simulink model "robot_portique_2_axes"  (R2024b)
settings: Solver=VariableStepAuto  StartTime=0.0  StopTime=21  RelTol=1e-3
settings Model: Creator=firas  LastModifiedBy=firas

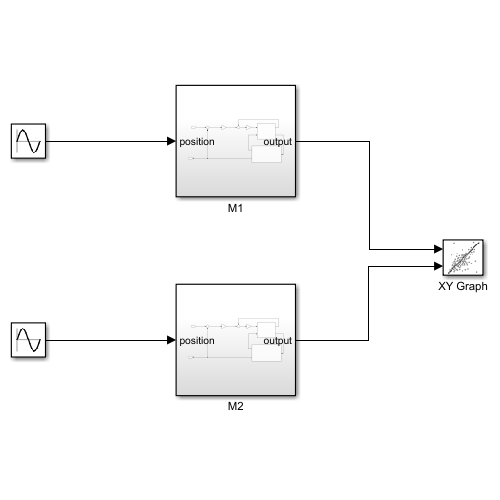
[thumbnail: Simulink's stored preview of the top-level diagram]
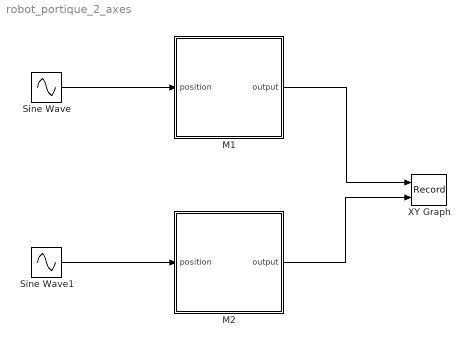
== system robot_portique_2_axes ==
  M1 : Subsystem
  M2 : Subsystem
  Sine Wave : Sin  Frequency=pi/10  Phase=pi/2  SampleTime=0
  Sine Wave1 : Sin  Frequency=pi/10  SampleTime=0
  XY Graph : Record  FileSettingsInternal="{\"entries\":[{\"content\":{\"excelSettings\":{\"content\":{},\"type\":\"Streamout.ExcelSettings\"}},\"type\":\"Streamout.FileSettingStorage\",\"uuid\":\"\"}],\"packageUris\":[\"http:\\/\\/schema.mathworks.com\\/mf0\\/streamout_blocks\\/R2020a\"],\"version\":\"1.0\"}"  Layout=[1 1]  SignalsInternal="{\"entries\":[{\"content\":{\"signals\":[{\"content\":{\"blockPath\":[],\"dimensions\":[1],\"domain\":\"\",\"lineColor\":\"#a2142f\",\"plots\":[ 1 ],\"port\":1,\"sid\":[\"\"],\"signalID\":1,\"signalName\":\"M1\"},\"type\":\"RecordBlkView.Signal\",\"uuid\":\"\"},{\"content\":{\"blockPath\":[],\"dimensions\":[1],\"domain\":\"\",\"lineColor\":\"#139fff\",\"plots\":[ 1 ],\"port\":2,\"sid\":[\"\"],\"signalID\":2,\"signalName\":\"M2\"},\"type\":\"RecordBlkView.Signal\",\"uuid\":\"\"}]},\"type\":\"RecordBlkView.InputSignals\",\"uuid\":\"\"}],\"packageUris\":[\"http:\\/\\/schema.mathworks.com\\/mf0\\/streamout_blocks\\/R2020a\"],\"version\":\"1.0\"}"  VisualizationBindings="{\"xyplotplugin\":{\"info\":[{\"series\":[{\"bindingParametersList\":[{\"parameter\":\"X-Axis\",\"signalID\":1,\"signalName\":\"M1\"},{\"parameter\":\"Y-Axis\",\"signalID\":2,\"signalName\":\"M2\"}],\"seriesID\":0}],\"subplotID\":1}]}}"  CompatibilityTag=XY
  wires:
  Sine Wave/1 -> M1/1(position)
  Sine Wave1/1 -> M2/1(position)
  M1/1(output) -> XY Graph/1
  M2/1(output) -> XY Graph/2

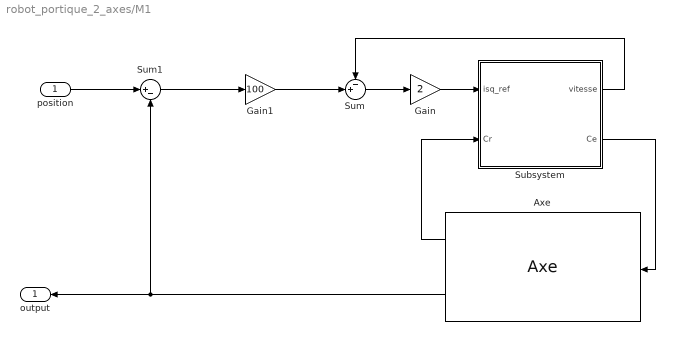
== system robot_portique_2_axes/M1 ==
  position : Inport
  Axe : S-Function  FunctionName=Axe  SFunctionModules=Axe_wrapper.c  SFunctionDeploymentMode=off  EnableBusSupport=off  mask(S-Function Builder){}
      mask help: Simulink:masks:SFunctionBuilder_MD
      mask init:
      | val = [[.9  0.75 0.75 1 1 .9 .9 1]',[1 1 0.75 0.75 .9 .9 1 .9]'];try , sys = get_param(gcb,'SfunBuilderFcnName');if isempty(sys), sys = get_param(gcb,'FunctionName'); end,catch, sys = get_param(gcb,'FunctionName'); end
      settings: CopyFcn=set_param(gcbh,'LinkStatus','none')  OpenFcn=sfunctionwizard(gcbh)
      mask Display:
      | plot(val(:,1),val(:,2))
      | disp(sys)
      | port_label('input',1,sprintf('%s', 'couple\_moteur'),'interpreter','tex')
      | port_label('output',1,sprintf('%s', 'couple\_resistant'),'interpreter','tex')
      | port_label('output',2,sprintf('%s', 'position'),'interpreter','tex')
  Gain : Gain  Gain=2
  Gain1 : Gain  Gain=100
  Subsystem : Subsystem
  Sum : Sum  Inputs=-+|
  Sum1 : Sum  Inputs=|+-
  output : Outport
  wires:
  Subsystem/1(vitesse) -> Sum/1
  Sum1/1 -> Gain1/1
  Axe/2 -> output/1, Sum1/2
  Gain1/1 -> Sum/2
  Subsystem/2(Ce) -> Axe/1
  Gain/1 -> Subsystem/1(isq_ref)
  Axe/1 -> Subsystem/2(Cr)
  Sum/1 -> Gain/1
  position/1 -> Sum1/1

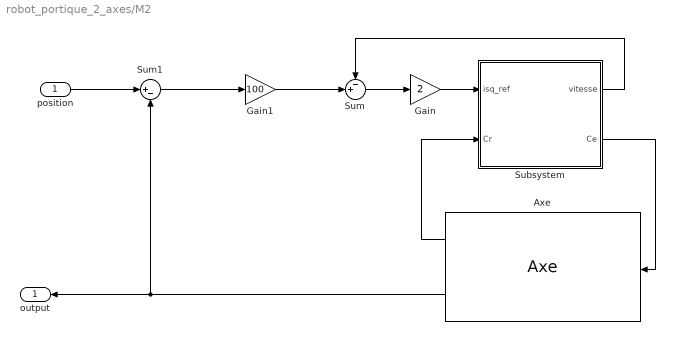
== system robot_portique_2_axes/M2 ==
  position : Inport
  Axe : S-Function  FunctionName=Axe  SFunctionModules=Axe_wrapper.c  SFunctionDeploymentMode=off  EnableBusSupport=off  mask(S-Function Builder){}
      mask help: Simulink:masks:SFunctionBuilder_MD
      mask init: same as robot_portique_2_axes/M1/Axe
      settings: CopyFcn=set_param(gcbh,'LinkStatus','none')  OpenFcn=sfunctionwizard(gcbh)
      mask Display:
      | plot(val(:,1),val(:,2))
      | disp(sys)
      | port_label('input',1,sprintf('%s', 'couple\_moteur'),'interpreter','tex')
      | port_label('output',1,sprintf('%s', 'couple\_resistant'),'interpreter','tex')
      | port_label('output',2,sprintf('%s', 'position'),'interpreter','tex')
  Gain : Gain  Gain=2
  Gain1 : Gain  Gain=100
  Subsystem : Subsystem
  Sum : Sum  Inputs=-+|
  Sum1 : Sum  Inputs=|+-
  output : Outport
  wires:
  position/1 -> Sum1/1
  Sum/1 -> Gain/1
  Axe/1 -> Subsystem/2(Cr)
  Gain/1 -> Subsystem/1(isq_ref)
  Subsystem/2(Ce) -> Axe/1
  Gain1/1 -> Sum/2
  Axe/2 -> Sum1/2, output/1
  Sum1/1 -> Gain1/1
  Subsystem/1(vitesse) -> Sum/1

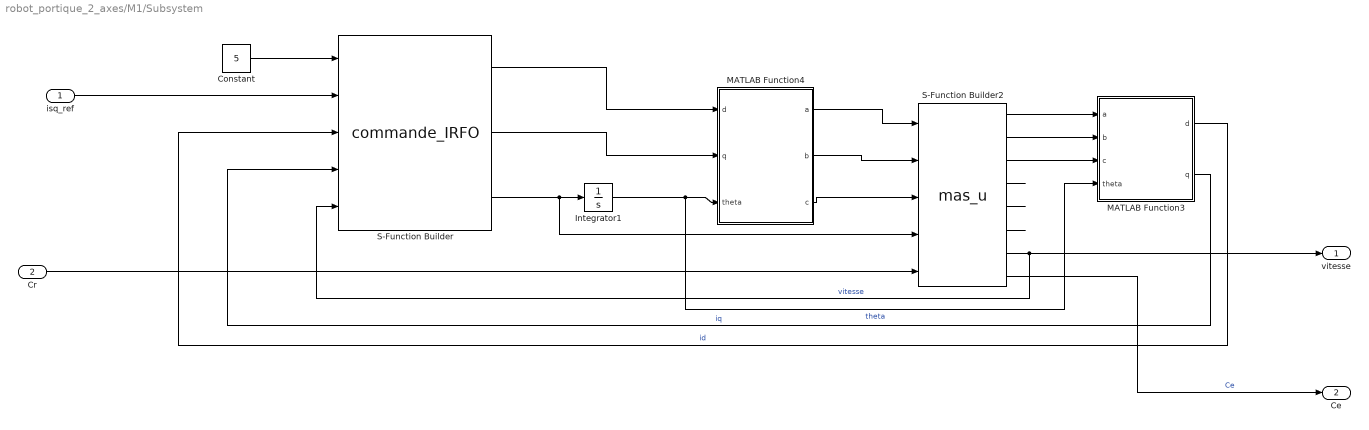
== system robot_portique_2_axes/M1/Subsystem ==
  isq_ref : Inport
  Cr : Inport  Port=2
  Constant : Constant  Value=5
  Integrator1 : Integrator
  MATLAB Function3 : MATLAB Function  TreatAsAtomicUnit=on
  MATLAB Function4 : MATLAB Function  TreatAsAtomicUnit=on
  S-Function Builder : S-Function  FunctionName=commande_IRFO  SFunctionModules=commande_IRFO_wrapper.c  SFunctionDeploymentMode=off  EnableBusSupport=off  mask(S-Function Builder){}
      mask help: Simulink:masks:SFunctionBuilder_MD
      mask init: same as robot_portique_2_axes/M1/Axe
      settings: CopyFcn=set_param(gcbh,'LinkStatus','none')  OpenFcn=sfunctionwizard(gcbh)
      mask Display:
      | plot(val(:,1),val(:,2))
      | disp(sys)
      | port_label('input',1,sprintf('%s', 'iphi\_ref'),'interpreter','tex')
      | port_label('input',2,sprintf('%s', 'isq\_ref'),'interpreter','tex')
      | port_label('input',3,sprintf('%s', 'isd'),'interpreter','tex')
      | port_label('input',4,sprintf('%s', 'isq'),'interpreter','tex')
      | port_label('input',5,sprintf('%s', 'vitesse'),'interpreter','tex')
      | port_label('output',1,sprintf('%s', 'vsd'),'interpreter','tex')
      | port_label('output',2,sprintf('%s', 'vsq'),'interpreter','tex')
      | port_label('output',3,sprintf('%s', 'ws'),'interpreter','tex')
  S-Function Builder2 : S-Function  FunctionName=mas_u  SFunctionModules=mas_u_wrapper.c  SFunctionDeploymentMode=off  EnableBusSupport=off  mask(S-Function Builder){}
      mask help: Simulink:masks:SFunctionBuilder_MD
      mask init: same as robot_portique_2_axes/M1/Axe
      settings: CopyFcn=set_param(gcbh,'LinkStatus','none')  OpenFcn=sfunctionwizard(gcbh)
      mask Display:
      | plot(val(:,1),val(:,2))
      | disp(sys)
      | port_label('input',1,sprintf('%s', 'vsa'),'interpreter','tex')
      | port_label('input',2,sprintf('%s', 'vsb'),'interpreter','tex')
      | port_label('input',3,sprintf('%s', 'vsc'),'interpreter','tex')
      | port_label('input',4,sprintf('%s', 'ws'),'interpreter','tex')
      | port_label('input',5,sprintf('%s', 'Cr'),'interpreter','tex')
      | port_label('output',1,sprintf('%s', 'isa'),'interpreter','tex')
      | port_label('output',2,sprintf('%s', 'isb'),'interpreter','tex')
      | port_label('output',3,sprintf('%s', 'isc'),'interpreter','tex')
      | port_label('output',4,sprintf('%s', 'ira'),'interpreter','tex')
      | port_label('output',5,sprintf('%s', 'irb'),'interpreter','tex')
      | port_label('output',6,sprintf('%s', 'irc'),'interpreter','tex')
      | port_label('output',7,sprintf('%s', 'vitesse'),'interpreter','tex')
      | port_label('output',8,sprintf('%s', 'Ce'),'interpreter','tex')
  vitesse : Outport
  Ce : Outport  Port=2
  wires:
  S-Function Builder2/4 -> ?
  S-Function Builder/2 -> MATLAB Function4/2(q)
  Integrator1/1 -> MATLAB Function4/3(theta), MATLAB Function3/4(theta)  "theta"
  S-Function Builder2/5 -> ?
  S-Function Builder/3 -> S-Function Builder2/4, Integrator1/1
  S-Function Builder2/1 -> MATLAB Function3/1(a)
  S-Function Builder2/7 -> vitesse/1, S-Function Builder/5  "vitesse"
  MATLAB Function3/1(d) -> S-Function Builder/3  "id"
  S-Function Builder2/2 -> MATLAB Function3/2(b)
  MATLAB Function4/1(a) -> S-Function Builder2/1
  S-Function Builder2/3 -> MATLAB Function3/3(c)
  Cr/1 -> S-Function Builder2/5
  MATLAB Function4/3(c) -> S-Function Builder2/3
  Constant/1 -> S-Function Builder/1
  S-Function Builder/1 -> MATLAB Function4/1(d)
  MATLAB Function3/2(q) -> S-Function Builder/4  "iq"
  MATLAB Function4/2(b) -> S-Function Builder2/2
  isq_ref/1 -> S-Function Builder/2
  S-Function Builder2/6 -> ?
  S-Function Builder2/8 -> Ce/1  "Ce"

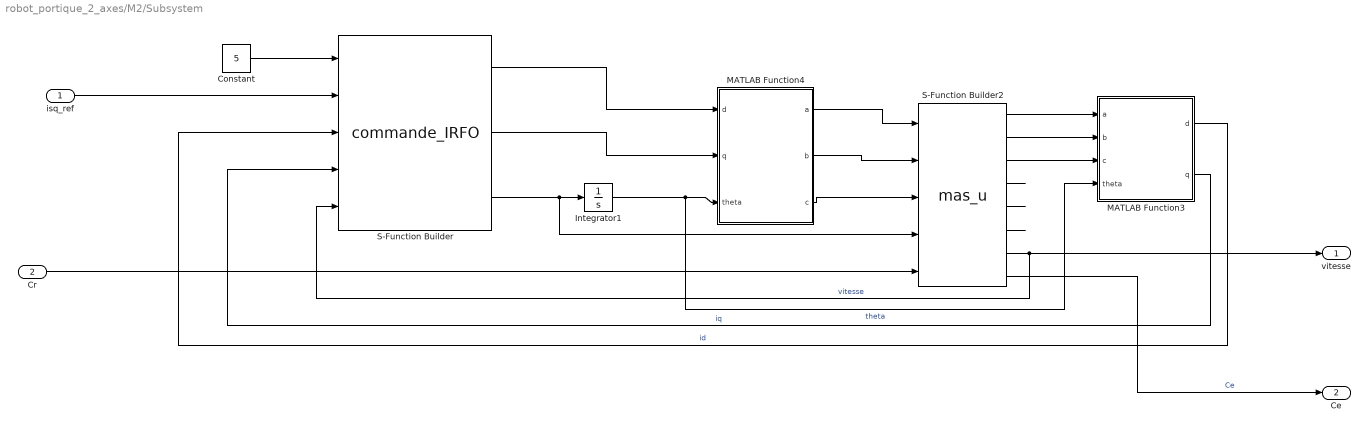
== system robot_portique_2_axes/M2/Subsystem ==
  isq_ref : Inport
  Cr : Inport  Port=2
  Constant : Constant  Value=5
  Integrator1 : Integrator
  MATLAB Function3 : MATLAB Function  TreatAsAtomicUnit=on
  MATLAB Function4 : MATLAB Function  TreatAsAtomicUnit=on
  S-Function Builder : S-Function  FunctionName=commande_IRFO  SFunctionModules=commande_IRFO_wrapper.c  SFunctionDeploymentMode=off  EnableBusSupport=off  mask(S-Function Builder){}
      mask help: Simulink:masks:SFunctionBuilder_MD
      mask init: same as robot_portique_2_axes/M1/Axe
      settings: CopyFcn=set_param(gcbh,'LinkStatus','none')  OpenFcn=sfunctionwizard(gcbh)
      mask Display:
      | plot(val(:,1),val(:,2))
      | disp(sys)
      | port_label('input',1,sprintf('%s', 'iphi\_ref'),'interpreter','tex')
      | port_label('input',2,sprintf('%s', 'isq\_ref'),'interpreter','tex')
      | port_label('input',3,sprintf('%s', 'isd'),'interpreter','tex')
      | port_label('input',4,sprintf('%s', 'isq'),'interpreter','tex')
      | port_label('input',5,sprintf('%s', 'vitesse'),'interpreter','tex')
      | port_label('output',1,sprintf('%s', 'vsd'),'interpreter','tex')
      | port_label('output',2,sprintf('%s', 'vsq'),'interpreter','tex')
      | port_label('output',3,sprintf('%s', 'ws'),'interpreter','tex')
  S-Function Builder2 : S-Function  FunctionName=mas_u  SFunctionModules=mas_u_wrapper.c  SFunctionDeploymentMode=off  EnableBusSupport=off  mask(S-Function Builder){}
      mask help: Simulink:masks:SFunctionBuilder_MD
      mask init: same as robot_portique_2_axes/M1/Axe
      settings: CopyFcn=set_param(gcbh,'LinkStatus','none')  OpenFcn=sfunctionwizard(gcbh)
      mask Display:
      | plot(val(:,1),val(:,2))
      | disp(sys)
      | port_label('input',1,sprintf('%s', 'vsa'),'interpreter','tex')
      | port_label('input',2,sprintf('%s', 'vsb'),'interpreter','tex')
      | port_label('input',3,sprintf('%s', 'vsc'),'interpreter','tex')
      | port_label('input',4,sprintf('%s', 'ws'),'interpreter','tex')
      | port_label('input',5,sprintf('%s', 'Cr'),'interpreter','tex')
      | port_label('output',1,sprintf('%s', 'isa'),'interpreter','tex')
      | port_label('output',2,sprintf('%s', 'isb'),'interpreter','tex')
      | port_label('output',3,sprintf('%s', 'isc'),'interpreter','tex')
      | port_label('output',4,sprintf('%s', 'ira'),'interpreter','tex')
      | port_label('output',5,sprintf('%s', 'irb'),'interpreter','tex')
      | port_label('output',6,sprintf('%s', 'irc'),'interpreter','tex')
      | port_label('output',7,sprintf('%s', 'vitesse'),'interpreter','tex')
      | port_label('output',8,sprintf('%s', 'Ce'),'interpreter','tex')
  vitesse : Outport
  Ce : Outport  Port=2
  wires:
  S-Function Builder2/8 -> Ce/1  "Ce"
  S-Function Builder2/6 -> ?
  isq_ref/1 -> S-Function Builder/2
  MATLAB Function4/2(b) -> S-Function Builder2/2
  MATLAB Function3/2(q) -> S-Function Builder/4  "iq"
  S-Function Builder/1 -> MATLAB Function4/1(d)
  Constant/1 -> S-Function Builder/1
  MATLAB Function4/3(c) -> S-Function Builder2/3
  Cr/1 -> S-Function Builder2/5
  S-Function Builder2/3 -> MATLAB Function3/3(c)
  MATLAB Function4/1(a) -> S-Function Builder2/1
  S-Function Builder2/2 -> MATLAB Function3/2(b)
  MATLAB Function3/1(d) -> S-Function Builder/3  "id"
  S-Function Builder2/7 -> S-Function Builder/5, vitesse/1  "vitesse"
  S-Function Builder2/1 -> MATLAB Function3/1(a)
  S-Function Builder/3 -> Integrator1/1, S-Function Builder2/4
  S-Function Builder2/5 -> ?
  Integrator1/1 -> MATLAB Function3/4(theta), MATLAB Function4/3(theta)  "theta"
  S-Function Builder/2 -> MATLAB Function4/2(q)
  S-Function Builder2/4 -> ?

== matlab function robot_portique_2_axes/M2/Subsystem/MATLAB Function3 ==
  data: a input; d output; b input; c input; theta input; q output
function [d,q] = Park_direct(a,b,c,theta)
    
     d = sqrt(2/3)*[cos(theta),cos(theta-2*pi/3),cos(theta+2*pi/3)]*[a;b;c];
     q = sqrt(2/3)*[-sin(theta),-sin(theta -2*pi/3),-sin(theta +2*pi/3)]*[a ; b ; c];
    
end

== matlab function robot_portique_2_axes/M2/Subsystem/MATLAB Function4 ==
  data: d input; a output; q input; theta input; b output; c output
function [a,b,c] = inverse_Park(d,q,theta)
    a = sqrt(2/3)*[cos(theta) -sin(theta)]*[d;q];
    b = sqrt(2/3)*[cos(theta-2*pi/3) -sin(theta-2*pi/3)]*[d;q];
    c = sqrt(2/3)*[cos(theta+2*pi/3) -sin(theta+2*pi/3)]*[d;q];
end

== matlab function robot_portique_2_axes/M1/Subsystem/MATLAB Function3 ==
  data: a input; d output; b input; c input; theta input; q output
function [d,q] = Park_direct(a,b,c,theta)
    
     d = sqrt(2/3)*[cos(theta),cos(theta-2*pi/3),cos(theta+2*pi/3)]*[a;b;c];
     q = sqrt(2/3)*[-sin(theta),-sin(theta -2*pi/3),-sin(theta +2*pi/3)]*[a ; b ; c];
    
end

== matlab function robot_portique_2_axes/M1/Subsystem/MATLAB Function4 ==
  data: d input; a output; q input; theta input; b output; c output
function [a,b,c] = inverse_Park(d,q,theta)
    a = sqrt(2/3)*[cos(theta) -sin(theta)]*[d;q];
    b = sqrt(2/3)*[cos(theta-2*pi/3) -sin(theta-2*pi/3)]*[d;q];
    c = sqrt(2/3)*[cos(theta+2*pi/3) -sin(theta+2*pi/3)]*[d;q];
end
